simulink model "Actormodel"  (R2018b)
(part 3 of 25)

  dotprod168/1 -> Mux/168
  "IW{1,1}(169,:)'"/1 -> dotprod169/1
  dotprod169/1 -> Mux/169
  "IW{1,1}(170,:)'"/1 -> dotprod170/1
  dotprod170/1 -> Mux/170
  "IW{1,1}(171,:)'"/1 -> dotprod171/1
  dotprod171/1 -> Mux/171
  "IW{1,1}(172,:)'"/1 -> dotprod172/1
  dotprod172/1 -> Mux/172
  "IW{1,1}(173,:)'"/1 -> dotprod173/1
  dotprod173/1 -> Mux/173
  "IW{1,1}(174,:)'"/1 -> dotprod174/1
  dotprod174/1 -> Mux/174
  "IW{1,1}(175,:)'"/1 -> dotprod175/1
  dotprod175/1 -> Mux/175
  "IW{1,1}(176,:)'"/1 -> dotprod176/1
  dotprod176/1 -> Mux/176
  "IW{1,1}(177,:)'"/1 -> dotprod177/1
  dotprod177/1 -> Mux/177
  "IW{1,1}(178,:)'"/1 -> dotprod178/1
  dotprod178/1 -> Mux/178
  "IW{1,1}(179,:)'"/1 -> dotprod179/1
  dotprod179/1 -> Mux/179
  "IW{1,1}(180,:)'"/1 -> dotprod180/1
  dotprod180/1 -> Mux/180
  "IW{1,1}(181,:)'"/1 -> dotprod181/1
  dotprod181/1 -> Mux/181
  "IW{1,1}(182,:)'"/1 -> dotprod182/1
  dotprod182/1 -> Mux/182
  "IW{1,1}(183,:)'"/1 -> dotprod183/1
  dotprod183/1 -> Mux/183
  "IW{1,1}(184,:)'"/1 -> dotprod184/1
  dotprod184/1 -> Mux/184
  "IW{1,1}(185,:)'"/1 -> dotprod185/1
  dotprod185/1 -> Mux/185
  "IW{1,1}(186,:)'"/1 -> dotprod186/1
  dotprod186/1 -> Mux/186
  "IW{1,1}(187,:)'"/1 -> dotprod187/1
  dotprod187/1 -> Mux/187
  "IW{1,1}(188,:)'"/1 -> dotprod188/1
  dotprod188/1 -> Mux/188
  "IW{1,1}(189,:)'"/1 -> dotprod189/1
  dotprod189/1 -> Mux/189
  "IW{1,1}(190,:)'"/1 -> dotprod190/1
  dotprod190/1 -> Mux/190
  "IW{1,1}(191,:)'"/1 -> dotprod191/1
  dotprod191/1 -> Mux/191
  "IW{1,1}(192,:)'"/1 -> dotprod192/1
  dotprod192/1 -> Mux/192
  "IW{1,1}(193,:)'"/1 -> dotprod193/1
  dotprod193/1 -> Mux/193
  "IW{1,1}(194,:)'"/1 -> dotprod194/1
  dotprod194/1 -> Mux/194
  "IW{1,1}(195,:)'"/1 -> dotprod195/1
  dotprod195/1 -> Mux/195
  "IW{1,1}(196,:)'"/1 -> dotprod196/1
  dotprod196/1 -> Mux/196
  "IW{1,1}(197,:)'"/1 -> dotprod197/1
  dotprod197/1 -> Mux/197
  "IW{1,1}(198,:)'"/1 -> dotprod198/1
  dotprod198/1 -> Mux/198
  "IW{1,1}(199,:)'"/1 -> dotprod199/1
  dotprod199/1 -> Mux/199
  "IW{1,1}(200,:)'"/1 -> dotprod200/1
  dotprod200/1 -> Mux/200
  "IW{1,1}(201,:)'"/1 -> dotprod201/1
  dotprod201/1 -> Mux/201
  "IW{1,1}(202,:)'"/1 -> dotprod202/1
  dotprod202/1 -> Mux/202
  "IW{1,1}(203,:)'"/1 -> dotprod203/1
  dotprod203/1 -> Mux/203
  "IW{1,1}(204,:)'"/1 -> dotprod204/1
  dotprod204/1 -> Mux/204
  "IW{1,1}(205,:)'"/1 -> dotprod205/1
  dotprod205/1 -> Mux/205
  "IW{1,1}(206,:)'"/1 -> dotprod206/1
  dotprod206/1 -> Mux/206
  "IW{1,1}(207,:)'"/1 -> dotprod207/1
  dotprod207/1 -> Mux/207
  "IW{1,1}(208,:)'"/1 -> dotprod208/1
  dotprod208/1 -> Mux/208
  "IW{1,1}(209,:)'"/1 -> dotprod209/1
  dotprod209/1 -> Mux/209
  "IW{1,1}(210,:)'"/1 -> dotprod210/1
  dotprod210/1 -> Mux/210
  "IW{1,1}(211,:)'"/1 -> dotprod211/1
  dotprod211/1 -> Mux/211
  "IW{1,1}(212,:)'"/1 -> dotprod212/1
  dotprod212/1 -> Mux/212
  "IW{1,1}(213,:)'"/1 -> dotprod213/1
  dotprod213/1 -> Mux/213
  "IW{1,1}(214,:)'"/1 -> dotprod214/1
  dotprod214/1 -> Mux/214
  "IW{1,1}(215,:)'"/1 -> dotprod215/1
  dotprod215/1 -> Mux/215
  "IW{1,1}(216,:)'"/1 -> dotprod216/1
  dotprod216/1 -> Mux/216
  "IW{1,1}(217,:)'"/1 -> dotprod217/1
  dotprod217/1 -> Mux/217
  "IW{1,1}(218,:)'"/1 -> dotprod218/1
  dotprod218/1 -> Mux/218
  "IW{1,1}(219,:)'"/1 -> dotprod219/1
  dotprod219/1 -> Mux/219
  "IW{1,1}(220,:)'"/1 -> dotprod220/1
  dotprod220/1 -> Mux/220
  "IW{1,1}(221,:)'"/1 -> dotprod221/1
  dotprod221/1 -> Mux/221
  "IW{1,1}(222,:)'"/1 -> dotprod222/1
  dotprod222/1 -> Mux/222
  "IW{1,1}(223,:)'"/1 -> dotprod223/1
  dotprod223/1 -> Mux/223
  "IW{1,1}(224,:)'"/1 -> dotprod224/1
  dotprod224/1 -> Mux/224
  "IW{1,1}(225,:)'"/1 -> dotprod225/1
  dotprod225/1 -> Mux/225
  "IW{1,1}(226,:)'"/1 -> dotprod226/1
  dotprod226/1 -> Mux/226
  "IW{1,1}(227,:)'"/1 -> dotprod227/1
  dotprod227/1 -> Mux/227
  "IW{1,1}(228,:)'"/1 -> dotprod228/1
  dotprod228/1 -> Mux/228
  "IW{1,1}(229,:)'"/1 -> dotprod229/1
  dotprod229/1 -> Mux/229
  "IW{1,1}(230,:)'"/1 -> dotprod230/1
  dotprod230/1 -> Mux/230
  "IW{1,1}(231,:)'"/1 -> dotprod231/1
  dotprod231/1 -> Mux/231
  "IW{1,1}(232,:)'"/1 -> dotprod232/1
  dotprod232/1 -> Mux/232
  "IW{1,1}(233,:)'"/1 -> dotprod233/1
  dotprod233/1 -> Mux/233
  "IW{1,1}(234,:)'"/1 -> dotprod234/1
  dotprod234/1 -> Mux/234
  "IW{1,1}(235,:)'"/1 -> dotprod235/1
  dotprod235/1 -> Mux/235
  "IW{1,1}(236,:)'"/1 -> dotprod236/1
  dotprod236/1 -> Mux/236
  "IW{1,1}(237,:)'"/1 -> dotprod237/1
  dotprod237/1 -> Mux/237
  "IW{1,1}(238,:)'"/1 -> dotprod238/1
  dotprod238/1 -> Mux/238
  "IW{1,1}(239,:)'"/1 -> dotprod239/1
  dotprod239/1 -> Mux/239
  "IW{1,1}(240,:)'"/1 -> dotprod240/1
  dotprod240/1 -> Mux/240
  "IW{1,1}(241,:)'"/1 -> dotprod241/1
  dotprod241/1 -> Mux/241
  "IW{1,1}(242,:)'"/1 -> dotprod242/1
  dotprod242/1 -> Mux/242
  "IW{1,1}(243,:)'"/1 -> dotprod243/1
  dotprod243/1 -> Mux/243
  "IW{1,1}(244,:)'"/1 -> dotprod244/1
  dotprod244/1 -> Mux/244
  "IW{1,1}(245,:)'"/1 -> dotprod245/1
  dotprod245/1 -> Mux/245
  "IW{1,1}(246,:)'"/1 -> dotprod246/1
  dotprod246/1 -> Mux/246
  "IW{1,1}(247,:)'"/1 -> dotprod247/1
  dotprod247/1 -> Mux/247
  "IW{1,1}(248,:)'"/1 -> dotprod248/1
  dotprod248/1 -> Mux/248
  "IW{1,1}(249,:)'"/1 -> dotprod249/1
  dotprod249/1 -> Mux/249
  "IW{1,1}(250,:)'"/1 -> dotprod250/1
  dotprod250/1 -> Mux/250
  "IW{1,1}(251,:)'"/1 -> dotprod251/1
  dotprod251/1 -> Mux/251
  "IW{1,1}(252,:)'"/1 -> dotprod252/1
  dotprod252/1 -> Mux/252
  "IW{1,1}(253,:)'"/1 -> dotprod253/1
  dotprod253/1 -> Mux/253
  "IW{1,1}(254,:)'"/1 -> dotprod254/1
  dotprod254/1 -> Mux/254
  "IW{1,1}(255,:)'"/1 -> dotprod255/1
  dotprod255/1 -> Mux/255
  "IW{1,1}(256,:)'"/1 -> dotprod256/1
  dotprod256/1 -> Mux/256
  "IW{1,1}(257,:)'"/1 -> dotprod257/1
  dotprod257/1 -> Mux/257
  "IW{1,1}(258,:)'"/1 -> dotprod258/1
  dotprod258/1 -> Mux/258
  "IW{1,1}(259,:)'"/1 -> dotprod259/1
  dotprod259/1 -> Mux/259
  "IW{1,1}(260,:)'"/1 -> dotprod260/1
  dotprod260/1 -> Mux/260
  "IW{1,1}(261,:)'"/1 -> dotprod261/1
  dotprod261/1 -> Mux/261
  "IW{1,1}(262,:)'"/1 -> dotprod262/1
  dotprod262/1 -> Mux/262
  "IW{1,1}(263,:)'"/1 -> dotprod263/1
  dotprod263/1 -> Mux/263
  "IW{1,1}(264,:)'"/1 -> dotprod264/1
  dotprod264/1 -> Mux/264
  "IW{1,1}(265,:)'"/1 -> dotprod265/1
  dotprod265/1 -> Mux/265
  "IW{1,1}(266,:)'"/1 -> dotprod266/1
  dotprod266/1 -> Mux/266
  "IW{1,1}(267,:)'"/1 -> dotprod267/1
  dotprod267/1 -> Mux/267
  "IW{1,1}(268,:)'"/1 -> dotprod268/1
  dotprod268/1 -> Mux/268
  "IW{1,1}(269,:)'"/1 -> dotprod269/1
  dotprod269/1 -> Mux/269
  "IW{1,1}(270,:)'"/1 -> dotprod270/1
  dotprod270/1 -> Mux/270
  "IW{1,1}(271,:)'"/1 -> dotprod271/1
  dotprod271/1 -> Mux/271
  "IW{1,1}(272,:)'"/1 -> dotprod272/1
  dotprod272/1 -> Mux/272
  "IW{1,1}(273,:)'"/1 -> dotprod273/1
  dotprod273/1 -> Mux/273
  "IW{1,1}(274,:)'"/1 -> dotprod274/1
  dotprod274/1 -> Mux/274
  "IW{1,1}(275,:)'"/1 -> dotprod275/1
  dotprod275/1 -> Mux/275
  "IW{1,1}(276,:)'"/1 -> dotprod276/1
  dotprod276/1 -> Mux/276
  "IW{1,1}(277,:)'"/1 -> dotprod277/1
  dotprod277/1 -> Mux/277
  "IW{1,1}(278,:)'"/1 -> dotprod278/1
  dotprod278/1 -> Mux/278
  "IW{1,1}(279,:)'"/1 -> dotprod279/1
  dotprod279/1 -> Mux/279
  "IW{1,1}(280,:)'"/1 -> dotprod280/1
  dotprod280/1 -> Mux/280
  "IW{1,1}(281,:)'"/1 -> dotprod281/1
  dotprod281/1 -> Mux/281
  "IW{1,1}(282,:)'"/1 -> dotprod282/1
  dotprod282/1 -> Mux/282
  "IW{1,1}(283,:)'"/1 -> dotprod283/1
  dotprod283/1 -> Mux/283
  "IW{1,1}(284,:)'"/1 -> dotprod284/1
  dotprod284/1 -> Mux/284
  "IW{1,1}(285,:)'"/1 -> dotprod285/1
  dotprod285/1 -> Mux/285
  "IW{1,1}(286,:)'"/1 -> dotprod286/1
  dotprod286/1 -> Mux/286
  "IW{1,1}(287,:)'"/1 -> dotprod287/1
  dotprod287/1 -> Mux/287
  "IW{1,1}(288,:)'"/1 -> dotprod288/1
  dotprod288/1 -> Mux/288
  "IW{1,1}(289,:)'"/1 -> dotprod289/1
  dotprod289/1 -> Mux/289
  "IW{1,1}(290,:)'"/1 -> dotprod290/1
  dotprod290/1 -> Mux/290
  "IW{1,1}(291,:)'"/1 -> dotprod291/1
  dotprod291/1 -> Mux/291
  "IW{1,1}(292,:)'"/1 -> dotprod292/1
  dotprod292/1 -> Mux/292
  "IW{1,1}(293,:)'"/1 -> dotprod293/1
  dotprod293/1 -> Mux/293
  "IW{1,1}(294,:)'"/1 -> dotprod294/1
  dotprod294/1 -> Mux/294
  "IW{1,1}(295,:)'"/1 -> dotprod295/1
  dotprod295/1 -> Mux/295
  "IW{1,1}(296,:)'"/1 -> dotprod296/1
  dotprod296/1 -> Mux/296
  "IW{1,1}(297,:)'"/1 -> dotprod297/1
  dotprod297/1 -> Mux/297
  "IW{1,1}(298,:)'"/1 -> dotprod298/1
  dotprod298/1 -> Mux/298
  "IW{1,1}(299,:)'"/1 -> dotprod299/1
  dotprod299/1 -> Mux/299
  "IW{1,1}(300,:)'"/1 -> dotprod300/1
  dotprod300/1 -> Mux/300
  Mux/1 -> "iz{1,1}"/1
